simulink library "lib_rate_limiter"  (R2023a)
settings: Solver=VariableStepAuto  StartTime=0.0  StopTime=10.0  RelTol=1e-3
undefined symbols (not defined in the file): parCharFreqFallSlewRate_s16n0b0, parCharFreqRiseSlewRate_s16n0b0, parMedTaskSampTime_u16d6b0, parSpdDrvtCharFreqMaxVal
libraries: lib_conversion x7, lib_resettable_unit_delay x1
settings Model: Creator=cav2ofo  LastModifiedBy=xiaoqiang.yuan
settings OptimizationCC: ReuseModelBlockBuffer=off

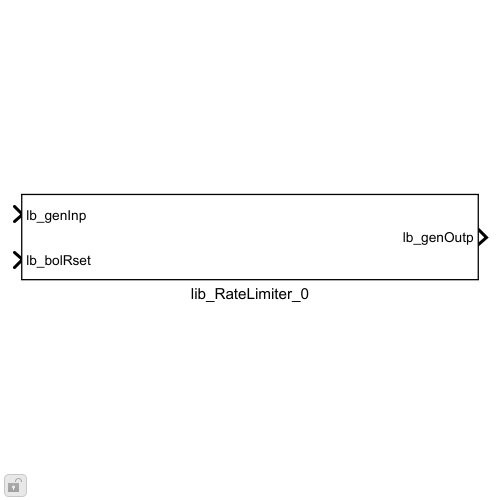
[thumbnail: Simulink's stored preview of the top-level diagram]
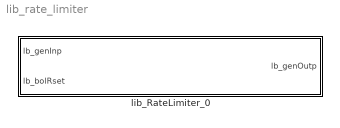
== system lib_rate_limiter ==
  lib_RateLimiter_0 : Subsystem  mask{lb_parSampTime=parMedTaskSampTime_u16d6b0, lb_parRiseSlewRate=parCharFreqRiseSlewRate_s16n0b0, lb_parFallSlewRate=parCharFreqFallSlewRate_s16n0b0, lb_parMaxInpVal=parSpdDrvtCharFreqMaxVal, lb_parMinInpVal=10}
      mask prompts: lb_parSampTime "Sampling time [s]:"; lb_parRiseSlewRate "Rising slew rate:"; lb_parFallSlewRate "Falling slew rate:"; lb_parMaxInpVal "Input signal max value"; lb_parMinInpVal "Input signal min value"
      mask init:
      | %Re-initialize parameters in Double
      | lb_parMaxInpVal = double(lb_parMaxInpVal);
      | lb_parMinInpVal = double(lb_parMinInpVal);
      | lb_parSampTime_temp = double(lb_parSampTime);
      | 
      | % Data type for input variation
      | lb_parInpVrntMaxVal = abs(lb_parMaxInpVal-lb_parMinInpVal);
      | 
      | % Data type for the derivative of the input signal
      | lb_parInpDrvtMaxVal = abs(lb_parMaxInpVal-lb_parMinInpVal)/lb_parSampTime_temp;
      | lb_parInpDrvtDataType = Simulink.NumericType;
      | lb_parInpDrvtDataType.DataTypeMode= 'Fixed-point: unspecified scaling';
      | if lb_parInpDrvtMaxVal <= (2^15)-1
      |     lb_parInpDrvtDataType.WordLength = 16;
      | else
      |     lb_parInpDrvtDataType.WordLength = 32;
      | end
      | 
      | %Min-Max limit for Sampling Time * Rise/Fall Slew rate 
      | lb_parAccmDataTypeMax = double(lb_parSampTime_temp*lb_parRiseSlewRate);
      | lb_parAccmDataTypeMin = double(lb_parSampTime_temp*lb_parFallSlewRate);
      | lb_parAccmDataType_temp = fi([lb_parAccmDataTypeMin lb_parAccmDataTypeMax]);
      | lb_parAccmDataType = Simulink.NumericType;
      | lb_parAccmDataType.DataTypeMode= 'Fixed-point: slope and bias scaling';
      | lb_parAccmDataType.Signedness = lb_parAccmDataType_temp.Signedness;
      | lb_parAccmDataType.WordLength = lb_parAccmDataType_temp.WordLength;
      | lb_parAccmDataType.Slope = 2^(-lb_parAccmDataType_temp.FractionLength);
      | 
      | % lb_parAccmDataType = Simulink.NumericType;
      | % lb_parAccmDataType.DataTypeMode= 'Fixed-point: unspecified scaling';
      | % if lb_parAccmDataTypeMax <= (2^15)-1
      | %     lb_parAccmDataType.WordLength = 16;
      | % else
      | %     lb_parAccmDataType.WordLength = 32;
      | % end
      | 
      | %% Convert to double parameters needed to compute data types
      | 
      | % lb_parRiseSlewRate = double(lb_parRiseSlewRate);
      | % 
      | % %% Define of data type for product u*Ts
      | % % lb_parIntgStepDataTypeMaxVal = lb_parMaxInpVal*lb_parSampTime*lb_parRiseSlewRate;
      | % lb_parOutpDataType = Simulink.NumericType;
      | % lb_parOutpDataType.DataTypeMode= 'Fixed-point: unspecified scaling';
      | % if lb_parMinInpVal < 0
      | %     lb_parOutpDataType.Signedness = 'Signed';
      | %     if lb_parMaxInpVal <= (2^16)/2-1
      | %         lb_parOutpDataType.WordLength = 16;
      | %     else
      | %         lb_parOutpDataType.WordLength = 32;
      | %     end
      | % else
      | %     lb_parOutpDataType.Signedness = 'Unsigned';
      | %         if lb_parMaxInpVal <= (2^16)-1
      | %         lb_parOutpDataType.WordLength = 16;
      | %     else
      | %         lb_parOutpDataType.WordLength = 32;
      | %     end
      | % end
      mask DialogControl DescGroupVar Prompt: Rate Limiter Block
      mask DialogControl DescTextVar Prompt: Rate Limiter Block

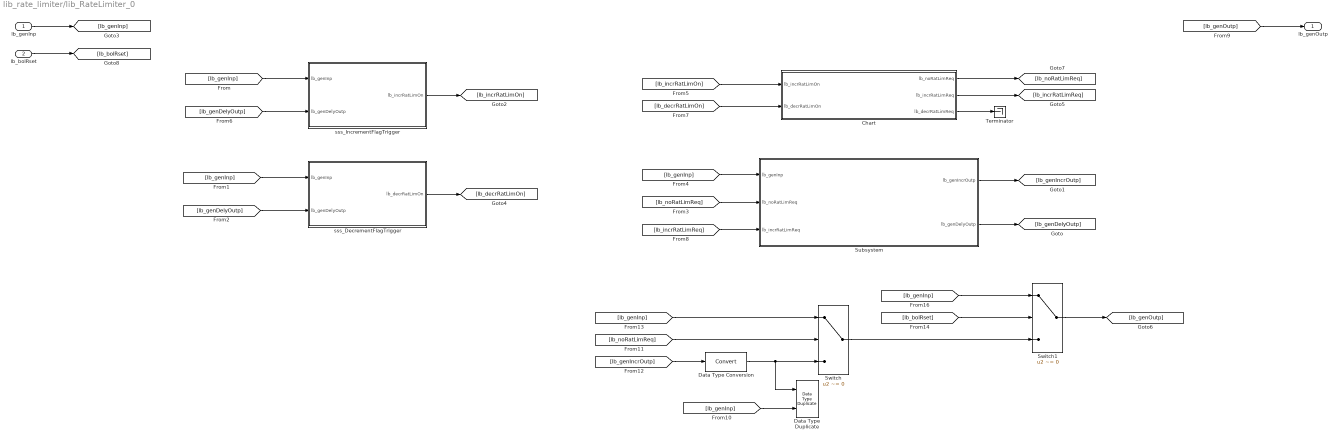
== system lib_rate_limiter/lib_RateLimiter_0 ==
  lb_genInp : Inport
  lb_bolRset : Inport  Port=2
  Chart : Stateflow chart  TreatAsAtomicUnit=on
  Data Type Duplicate : DataTypeDuplicate
  Data Type Conversion : DataTypeConversion  SaturateOnIntegerOverflow=off  RndMeth=Floor
  Subsystem : Subsystem
  Switch : Switch  Criteria=u2 ~= 0  SaturateOnIntegerOverflow=off  InputSameDT=off
  Switch1 : Switch  Criteria=u2 ~= 0  SaturateOnIntegerOverflow=off  InputSameDT=off
  Terminator : Terminator
  sss_DecrementFlagTrigger : Subsystem
  sss_IncrementFlagTrigger : Subsystem
  lb_genOutp : Outport
  wires:
  Switch1/1 -> [lb_genOutp]
  [lb_genInp] -> Switch1/1
  Switch/1 -> Switch1/3
  [lb_bolRset] -> Switch1/2
  lb_bolRset/1 -> [lb_bolRset]
  [lb_genInp] -> Switch/1
  [lb_noRatLimReq] -> Switch/2
  [lb_genInp] -> Data Type Duplicate/2
  Data Type Conversion/1 -> Switch/3, Data Type Duplicate/1
  [lb_genIncrOutp] -> Data Type Conversion/1
  [lb_noRatLimReq] -> Subsystem/2(lb_noRatLimReq)
  [lb_incrRatLimReq] -> Subsystem/3(lb_incrRatLimReq)
  [lb_genDelyOutp] -> sss_IncrementFlagTrigger/2(lb_genDelyOutp)
  Subsystem/2(lb_genDelyOutp) -> [lb_genDelyOutp]
  [lb_genOutp] -> lb_genOutp/1
  Subsystem/1(lb_genIncrOutp) -> [lb_genIncrOutp]
  [lb_genInp] -> Subsystem/1(lb_genInp)
  Chart/3(lb_decrRatLimReq) -> Terminator/1
  Chart/2(lb_incrRatLimReq) -> [lb_incrRatLimReq]
  Chart/1(lb_noRatLimReq) -> [lb_noRatLimReq]
  [lb_decrRatLimOn] -> Chart/2(lb_decrRatLimOn)
  [lb_incrRatLimOn] -> Chart/1(lb_incrRatLimOn)
  [lb_genInp] -> sss_DecrementFlagTrigger/1(lb_genInp)
  [lb_genDelyOutp] -> sss_DecrementFlagTrigger/2(lb_genDelyOutp)
  sss_DecrementFlagTrigger/1(lb_decrRatLimOn) -> [lb_decrRatLimOn]
  sss_IncrementFlagTrigger/1(lb_incrRatLimOn) -> [lb_incrRatLimOn]
  [lb_genInp] -> sss_IncrementFlagTrigger/1(lb_genInp)
  lb_genInp/1 -> [lb_genInp]

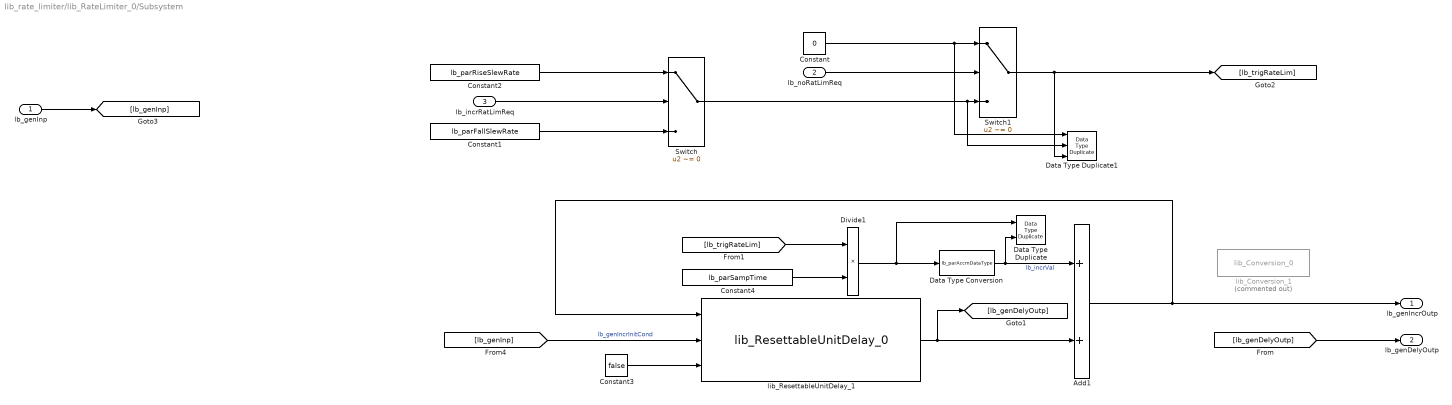
== system lib_rate_limiter/lib_RateLimiter_0/Subsystem ==
  lb_genInp : Inport
  lb_noRatLimReq : Inport  Port=2
  lb_incrRatLimReq : Inport  Port=3
  Add1 : Sum  OutDataTypeStr=Inherit: Inherit via back propagation  RndMeth=Simplest
  Constant : Constant  Value=0  OutDataTypeStr=Inherit: Inherit via back propagation  LockScale=on
  Constant1 : Constant  Value=lb_parFallSlewRate
  Constant2 : Constant  Value=lb_parRiseSlewRate
  Constant3 : Constant  Value=false  OutDataTypeStr=boolean
  Constant4 : Constant  Value=lb_parSampTime
  Data Type Duplicate : DataTypeDuplicate
  Data Type Duplicate1 : DataTypeDuplicate  NumInputPorts=3
  Data Type Conversion : DataTypeConversion  OutDataTypeStr=lb_parAccmDataType  RndMeth=Simplest  SaturateOnIntegerOverflow=off
  Divide1 : Product  Inputs=**  OutDataTypeStr=Inherit: Inherit via back propagation  RndMeth=Simplest
  Switch : Switch  Criteria=u2 ~= 0  SaturateOnIntegerOverflow=off  InputSameDT=off
  Switch1 : Switch  Criteria=u2 ~= 0  OutDataTypeStr=Inherit: Inherit via back propagation  SaturateOnIntegerOverflow=off  InputSameDT=off
  lib_Conversion_1 : lib_conversion/lib_Conversion_0  Commented=on  lb_parDataType=fixdt(1,16)  lb_parOutpMaxVal=lb_parMaxInpVal  lb_parOutpMinVal=lb_parMinInpVal  lb_parSatFlag=off
  lib_ResettableUnitDelay_1 : lib_resettable_unit_delay/lib_ResettableUnitDelay_0
  lb_genIncrOutp : Outport
  lb_genDelyOutp : Outport  Port=2
  wires:
  [lb_genInp] -> lib_ResettableUnitDelay_1/2  "lb_genIncrInitCond"
  Add1/1 -> lb_genIncrOutp/1, lib_ResettableUnitDelay_1/1
  lib_ResettableUnitDelay_1/1 -> [lb_genDelyOutp], Add1/2
  Data Type Conversion/1 -> Data Type Duplicate/2, Add1/1  "lb_incrVal"
  [lb_trigRateLim] -> Divide1/1
  Constant1/1 -> Switch/3
  Switch1/1 -> [lb_trigRateLim], Data Type Duplicate1/3
  Constant2/1 -> Switch/1
  Switch/1 -> Switch1/3, Data Type Duplicate1/2
  Constant/1 -> Switch1/1, Data Type Duplicate1/1
  lb_incrRatLimReq/1 -> Switch/2
  lb_noRatLimReq/1 -> Switch1/2
  Constant3/1 -> lib_ResettableUnitDelay_1/3
  Divide1/1 -> Data Type Duplicate/1, Data Type Conversion/1
  Constant4/1 -> Divide1/2
  lb_genInp/1 -> [lb_genInp]
  [lb_genDelyOutp] -> lb_genDelyOutp/1

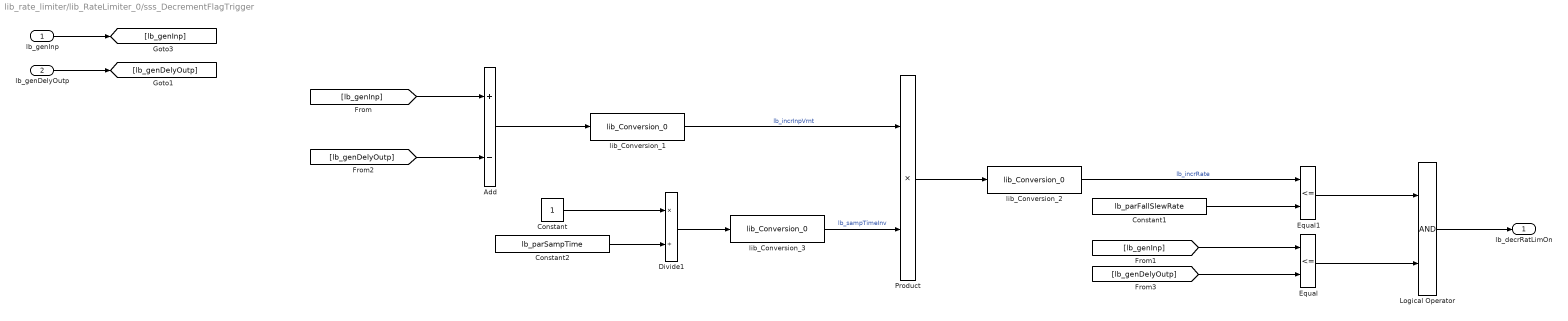
== system lib_rate_limiter/lib_RateLimiter_0/sss_DecrementFlagTrigger ==
  lb_genInp : Inport
  lb_genDelyOutp : Inport  Port=2
  Add : Sum  Inputs=+-  OutDataTypeStr=Inherit: Inherit via back propagation  RndMeth=Simplest
  Constant : Constant  OutDataTypeStr=uint16
  Constant1 : Constant  Value=lb_parFallSlewRate
  Constant2 : Constant  Value=lb_parSampTime
  Divide1 : Product  Inputs=*/  OutDataTypeStr=Inherit: Inherit via back propagation  RndMeth=Simplest
  Equal : RelationalOperator  Operator=<=  OutDataTypeStr=boolean  RndMeth=Simplest  InputSameDT=off
  Equal1 : RelationalOperator  Operator=<=  OutDataTypeStr=boolean  RndMeth=Simplest  InputSameDT=off
  Logical Operator : Logic  AllPortsSameDT=off  OutDataTypeStr=boolean
  Product : Product  OutDataTypeStr=Inherit: Inherit via back propagation
  lib_Conversion_1 : lib_conversion/lib_Conversion_0  lb_parDataType=fixdt(1,32)  lb_parOutpMaxVal=lb_parInpVrntMaxVal  lb_parOutpMinVal=[]  lb_parSatFlag=off
  lib_Conversion_2 : lib_conversion/lib_Conversion_0  lb_parDataType=lb_parInpDrvtDataType  lb_parOutpMaxVal=lb_parInpDrvtMaxVal  lb_parOutpMinVal=[]  lb_parSatFlag=off
  lib_Conversion_3 : lib_conversion/lib_Conversion_0  lb_parDataType=fixdt(0,32)  lb_parOutpMaxVal=1/double(lb_parSampTime)  lb_parOutpMinVal=[]  lb_parSatFlag=off
  lb_decrRatLimOn : Outport
  wires:
  lib_Conversion_3/1 -> Product/2  "lb_sampTimeInv"
  Divide1/1 -> lib_Conversion_3/1
  Constant2/1 -> Divide1/2
  Constant/1 -> Divide1/1
  lib_Conversion_1/1 -> Product/1  "lb_incrInpVrnt"
  Add/1 -> lib_Conversion_1/1
  [lb_genInp] -> Add/1
  lib_Conversion_2/1 -> Equal1/1  "lb_incrRate"
  [lb_genDelyOutp] -> Equal/2
  [lb_genDelyOutp] -> Add/2
  Constant1/1 -> Equal1/2
  lb_genDelyOutp/1 -> [lb_genDelyOutp]
  lb_genInp/1 -> [lb_genInp]
  Logical Operator/1 -> lb_decrRatLimOn/1
  Equal1/1 -> Logical Operator/1
  Product/1 -> lib_Conversion_2/1
  Equal/1 -> Logical Operator/2
  [lb_genInp] -> Equal/1

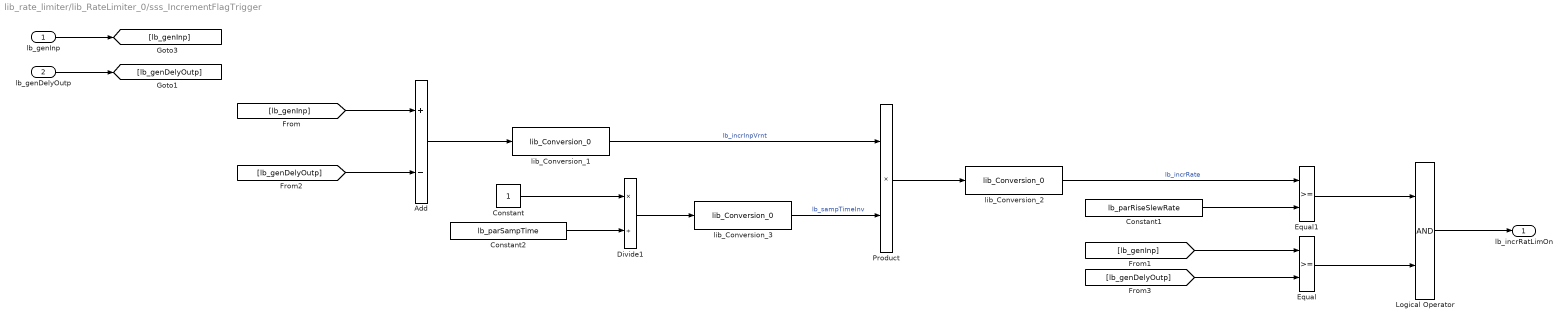
== system lib_rate_limiter/lib_RateLimiter_0/sss_IncrementFlagTrigger ==
  lb_genInp : Inport
  lb_genDelyOutp : Inport  Port=2
  Add : Sum  Inputs=+-  OutDataTypeStr=Inherit: Inherit via back propagation  RndMeth=Simplest
  Constant : Constant  OutDataTypeStr=uint16
  Constant1 : Constant  Value=lb_parRiseSlewRate
  Constant2 : Constant  Value=lb_parSampTime
  Divide1 : Product  Inputs=*/  OutDataTypeStr=Inherit: Inherit via back propagation  RndMeth=Simplest
  Equal : RelationalOperator  OutDataTypeStr=boolean  RndMeth=Simplest  InputSameDT=off
  Equal1 : RelationalOperator  OutDataTypeStr=boolean  RndMeth=Simplest  InputSameDT=off
  Logical Operator : Logic  AllPortsSameDT=off  OutDataTypeStr=boolean
  Product : Product  OutDataTypeStr=Inherit: Inherit via back propagation
  lib_Conversion_1 : lib_conversion/lib_Conversion_0  lb_parDataType=fixdt(1,32)  lb_parOutpMaxVal=lb_parInpVrntMaxVal  lb_parOutpMinVal=[]  lb_parSatFlag=off
  lib_Conversion_2 : lib_conversion/lib_Conversion_0  lb_parDataType=lb_parInpDrvtDataType  lb_parOutpMaxVal=lb_parInpDrvtMaxVal  lb_parOutpMinVal=[]  lb_parSatFlag=off
  lib_Conversion_3 : lib_conversion/lib_Conversion_0  lb_parDataType=fixdt(0,32)  lb_parOutpMaxVal=1/double(lb_parSampTime)  lb_parOutpMinVal=[]  lb_parSatFlag=off
  lb_incrRatLimOn : Outport
  wires:
  lib_Conversion_3/1 -> Product/2  "lb_sampTimeInv"
  Constant/1 -> Divide1/1
  Constant2/1 -> Divide1/2
  Divide1/1 -> lib_Conversion_3/1
  lib_Conversion_1/1 -> Product/1  "lb_incrInpVrnt"
  [lb_genInp] -> Add/1
  lib_Conversion_2/1 -> Equal1/1  "lb_incrRate"
  [lb_genDelyOutp] -> Equal/2
  [lb_genDelyOutp] -> Add/2
  Constant1/1 -> Equal1/2
  Product/1 -> lib_Conversion_2/1
  lb_genDelyOutp/1 -> [lb_genDelyOutp]
  lb_genInp/1 -> [lb_genInp]
  Logical Operator/1 -> lb_incrRatLimOn/1
  Equal1/1 -> Logical Operator/1
  Equal/1 -> Logical Operator/2
  [lb_genInp] -> Equal/1
  Add/1 -> lib_Conversion_1/1

== stateflow chart lib_rate_limiter/lib_RateLimiter_0/Chart ==
  (default) -> (junction 26)
  (junction 26) -> (junction 30) [order 1] : [~lb_incrRatLimOn  && lb_decrRatLimOn]
  (junction 26) -> (junction 1) [order 2]
  (junction 30) -> (junction 32) : {lb_noRatLimReq = false;
      | lb_incrRatLimReq = false;
      | lb_decrRatLimReq = true;}
  (junction 1) -> (junction 4) [order 1] : [lb_incrRatLimOn  && ~lb_decrRatLimOn]
  (junction 1) -> (junction 3) [order 2] : {lb_noRatLimReq = true;
      | lb_incrRatLimReq = false;
      | lb_decrRatLimReq = false;}
  (junction 4) -> (junction 6) : {lb_noRatLimReq = false;
      | lb_incrRatLimReq = true;
      | lb_decrRatLimReq = false;}
  (junction 6) -> (junction 3)
  (junction 3) -> (junction 28)
  (junction 32) -> (junction 28)
  (junction 28) -> (junction 38)
  data: lb_incrRatLimOn input boolean; lb_decrRatLimOn input boolean; lb_noRatLimReq output boolean; lb_incrRatLimReq output boolean; lb_decrRatLimReq output boolean
